simulink library "lib_AirProps_SpecificHeatConstVol"  (R2015a)
settings: Solver=ode45  StartTime=0.0  StopTime=10.0  RelTol=1e-3
settings Model: Creator=jlkratz  LastModifiedBy=jlkratz

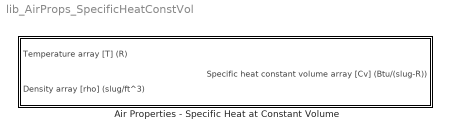
== system lib_AirProps_SpecificHeatConstVol ==
  Air Properties - Specific Heat at Constant Volume : Subsystem  mask(TSAT: Air Properties - Specific Heat at Constant Volume Block){BN_M=double(gcb)}
      mask prompts: BN_M "Block name"
      mask help:
      | This function provides an estimate of the specific heat at constant volume of air given its temperature and denisty. The function uses empirical relations which are valid for dry air in the temperature range of 60K - 2000K (108R - 3600R) and pressures up to 2000MPa. See the block help menu for details. This function is capable of evaluating the constant volume specific heat for various temperature and density combinations at the same time given 1-D arrays of consistent lengths for both the temperature and density inputs.
      |
      | Units are clearly stated on the inport and outport so assure that your inputs are in the specified units and the output is properly converted to your desired units after the calculation.
      mask Help: web(which('AirProps_TSAT_SpecificHeatConstVol.html'),'-helpbrowser')

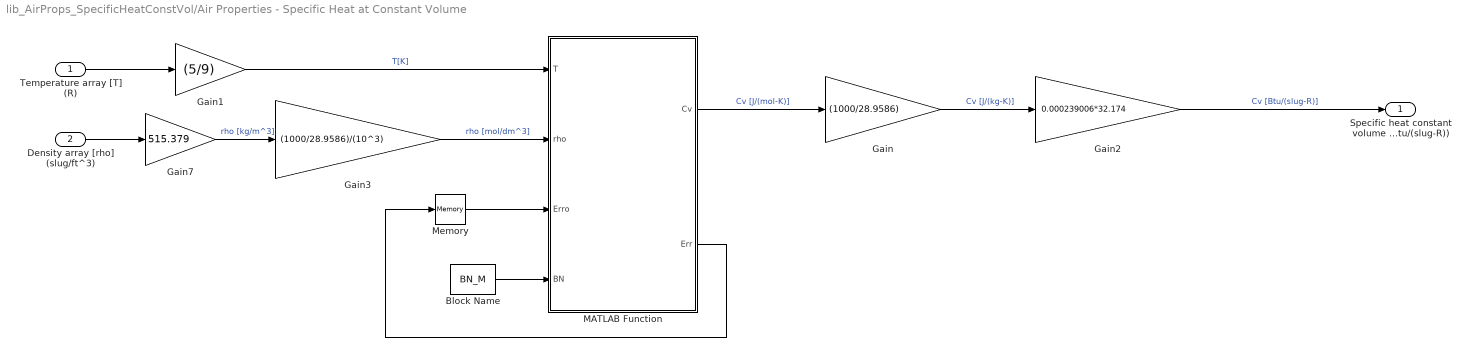
== system lib_AirProps_SpecificHeatConstVol/Air Properties - Specific Heat at Constant Volume ==
  Temperature array [T] (R) : Inport
  Density array [rho] (slug/ft^3) : Inport  Port=2
  Block Name : Constant  Value=BN_M
  Gain : Gain  Gain=(1000/28.9586)
  Gain1 : Gain  Gain=(5/9)
  Gain2 : Gain  Gain=0.000239006*32.174
  Gain3 : Gain  Gain=(1000/28.9586)/(10^3)
  Gain7 : Gain  Gain=515.379
  MATLAB Function : MATLAB Function  TreatAsAtomicUnit=on
  Memory : Memory  X0=zeros(1,3)
  Specific heat constant volume array [Cv] (Btu/(slug-R)) : Outport
  wires:
  Density array [rho] (slug/ft^3)/1 -> Gain7/1
  Gain7/1 -> Gain3/1  "rho [kg/m^3]"
  Gain3/1 -> MATLAB Function/2(rho)  "rho [mol/dm^3]"
  Block Name/1 -> MATLAB Function/4(BN)
  MATLAB Function/2(Err) -> Memory/1
  Memory/1 -> MATLAB Function/3(Erro)
  Gain/1 -> Gain2/1  "Cv [J/(kg-K)]"
  Gain1/1 -> MATLAB Function/1(T)  "T[K]"
  Gain2/1 -> Specific heat constant volume array [Cv] (Btu/(slug-R))/1  "Cv [Btu/(slug-R)]"
  Temperature array [T] (R)/1 -> Gain1/1
  MATLAB Function/1(Cv) -> Gain/1  "Cv [J/(mol-K)]"

== matlab function lib_AirProps_SpecificHeatConstVol/Air Properties - Specific Heat at Constant Volume/MATLAB Function ==
  data: T input; rho input; Cv output; Erro input; BN input; Err output
function [Cv,Err] = SpecificHeatConstVol_Air(T,rho,Erro,BN)
%#codegen

%Written By: Jonathan Kratz, NASA GRC
%Date: August 18, 2016
%Descirption: This function calculates the constant volume specifity heat 
%of air using empirical correlations from:
%   Lemmon, E., Jacobsen, R., Penoncello, S., and Friend, D., 
%   Thermodynamic Properties of Air and Mixtures of Nitrogen, Argon, and 
%   Oxygen From 60 to 2000K at pressure to 2000MPa,” Journal of Physics 
%   Chemistry Reference Data, Vol. 29, No. 3, 2000
%
%Inputs:
%   T - Temperature array of the air in Kelvin (K)
%   rho - Density array of the air (mol/dm^3)
%
%Outputs:
%   Cv - Specific heat constant volume array corresponding to T (J/(mol-K)) 

%Number of element is T to solve for Cp
n = length(T);
m = length(rho);
Cp = zeros(1,n);
Cv = zeros(1,n);
dalphar_ddel = zeros(1,n);
d2alphar_ddel2 = zeros(1,n);
d2alphar_ddeldtau = zeros(1,n);

%error checking
Err = Erro;
ErrNum = 1;
if n ~= m && Erro(ErrNum) == 0
    Err(ErrNum) = 1;
    fprintf('warning in %s: The input arrays T and rho must be the same length.\n',char(BN));
end
if min(T) < 60 && Erro(ErrNum) == 0
    Err(ErrNum) = 1;
    fprintf('warning in %s: At least 1 element of the temperature array is below the temperature range (60-2000K, 108-3600R) which the empirical correlation is valid\n',char(BN));
end
ErrNum = ErrNum + 1;
if max(T) > 2000 && Erro(ErrNum) == 0
    Err(ErrNum) = 1;
    fprintf('warning in %s: At least 1 element of the temperature array is above the temperature range (60-2000K, 108-3600R) which the empirical correlation is valid\n',char(BN));
end

%parameters
Tc = 132.6312; %K
rhoc = 10.4477; %mol-dm^-3
R = 8.314510; %universal gas constant J/(mol-K)

%calculate Helmholtz deriviatives ----------------------------------------%

%Coefficients and exponents for the equation of state for air
N = [0.118160747229, 0.713116392079, -1.61824192067, 0.0714140178971, -0.0865421396646, 0.134211176704, 0.0112626704218, -0.0420533228842, 0.0349008431982, 0.000164957183186, -0.101365037921, -0.173813690970, -0.0472103183731, -0.0122523554253, -0.146629609713, -0.0316055879821, 0.000233594806142, 0.0148287891978, -0.00938782884667];
i = [1.0, 1.0, 1.0, 2.0, 3.0, 3.0, 4.0, 4.0, 4.0, 6.0, 1.0, 3.0, 5.0, 6.0, 1.0, 3.0, 11.0, 1.0, 3.0];
j = [0.0, 0.33, 1.01, 0.0, 0.0, 0.15, 0.0, 0.2, 0.35, 1.35, 1.6, 0.8, 0.95, 1.25, 3.6, 6.0, 3.25, 3.5, 15.0];
l = [0.0, 0.0, 0.0, 0.0, 0.0, 0.0, 0.0, 0.0, 0.0, 0.0, 1.0, 1.0, 1.0, 1.0, 2.0, 2.0, 2.0, 3.0, 3.0];

%First derivative of residual Helmholtz energy with respect to rho/rhoc
for a = 1:n
    sum1 = 0;
    for k = 1:10
        sum1 = sum1 + i(k)*N(k)*(rho(a)/rhoc)^(i(k)-1)*(Tc/T(a))^j(k);
    end
    sum2 = 0;
    for k = 11:19
        sum2 = sum2 + i(k)*N(k)*(rho(a)/rhoc)^(i(k)-1)*(Tc/T(a))^j(k)*exp((rho(a)/rhoc)^l(k))*(i(k)-l(k)*(rho(a)/rhoc)^l(k));
    end
    dalphar_ddel(a) = sum1 + sum2;
end

%Second derivative of residual Helmholtz energy with respect to rho/rhoc
for a = 1:n
    sum1 = 0;
    for k = 1:10
        sum1 = sum1 + i(k)*(i(k)-1)*N(k)*(rho(a)/rhoc)^(i(k)-2)*(Tc/T(a))^j(k);
    end
    sum2 = 0;
    for k = 11:19
        sum2 = sum2 + N(k)*(rho(a)/rhoc)^(i(k)-2)*(Tc/T(a))^j(k)*exp(-(rho(a)/rhoc)^l(k))*((i(k)-l(k)*(rho(a)/rhoc)^l(k))*(i(k)-1-l(k)*(rho(a)/rhoc)^l(k))-l(k)^2*(rho(a)/rhoc)^l(k));
    end
    d2alphar_ddel2(a) = sum1 + sum2;
end

%Mixed derivative of residual Helmholtz energy
for a = 1:n
    sum1 = 0;
    for k = 1:10
        sum1 = sum1 + i(k)*j(k)*N(k)*(rho(a)/rhoc)^(i(k)-1)*(Tc/T(a))^(j(k)-1);
    end
    sum2 = 0;
    for k = 11:19
        sum2 = sum2 + j(k)*N(k)*(rho(a)/rhoc)^(i(k)-1)*(Tc/T(a))^(j(k)-1)*exp(-(rho(a)/rhoc)^l(k))*(i(k)-l(k)*(rho(a)/rhoc)^l(k));
    end
    d2alphar_ddeldtau(a) = sum1 + sum2;
end

%calculate heat capacity (Cp) --------------------------------------------%

%Coefficients of ideal gas expressions
N = [3.490888032, 2.395525583e-6, 7.172111248e-9, -3.115413101e-13, 0.223806688, 0.791309509, 0.212236768, 0.197938904, 3364.011, 2242.45, 11580.4];

for i = 1:n
    %Simplification variables
    u = N(9)/T(i);
    v = N(10)/T(i);
    w = N(11)/T(i);
    %Calculation of Cp (J/mol-K)
    sum = 0;
    for j = 1:4
        sum = sum + N(j)*T(i)^(j-1);
    end
    Cp(i) = R*(sum + N(5)/T(i)^1.5 + (N(6)*u^2.0*exp(u))/(exp(u)-1)^2.0 + (N(7)*v^2.0*exp(v))/((exp(v)-1)^2.0) + ((2.0/3.0)*N(8)*w^2.0*exp(-w))/((2.0/3.0)*exp(-w)+1)^2.0);
end

%calculate the heat capacity at constant volume (Cv) ---------------------%

%Cv (J/mol-K)
for i = 1:n
    Cv(i) = Cp(i) - R * ( (1 + (rho(i)/rhoc)*dalphar_ddel(i) - (rho(i)/rhoc)*(Tc/T(i))*d2alphar_ddeldtau(i))^2 / (1 + 2*(rho(i)/rhoc)*dalphar_ddel(i) + (rho(i)/rhoc)^2*d2alphar_ddel2(i)) );
end
